simulink model "motor_param_persist"  (R2021a)
settings: configuration reference "motor_ctrl_config" (kept outside this file)
model workspace (MAT data in the model file):
  debounce = 4
  debounce_cnt_def = Simulink.Parameter
  debounce_cnt_def.Value = 0
  debounce_cnt_def.DataType = 'int16'
  debounce_cnt_def.Dimensions = [1 1]
values from neighbouring files (symbols this model uses):
  ee_ram = 1    [motor_ctrl_data.sldd]
undefined symbols (not defined in the file or in its folder): ee_commit
libraries: simulink x1
settings Model: DataDictionary=motor_ctrl_data.sldd  ParameterArgumentNames=debounce_cnt_def  OrderedModelArguments=off  Creator=Litao  LastModifiedBy=Litao
settings ConfigSetRef: SourceName=motor_ctrl_config

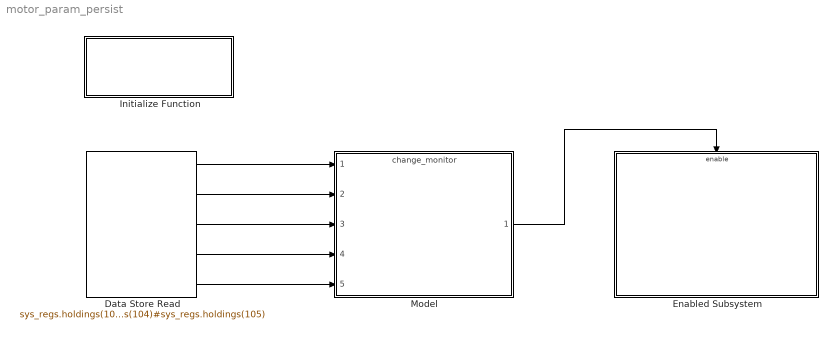
== system motor_param_persist ==
  Data Store Read : DataStoreRead  DataStoreName=sys_regs  DataStoreElements=sys_regs.holdings(101)#sys_regs.holdings(102)#sys_regs.holdings(103)#sys_regs.holdings(104)#sys_regs.holdings(105)  IndexOptions=Index vector (dialog)  Indices=1  OutputSizes=1
  Enabled Subsystem : Subsystem  TreatAsAtomicUnit=on
  Initialize Function : Subsystem  TreatAsAtomicUnit=on
  Model : ModelReference  ModelNameDialog=change_monitor.slx  SimulationMode=Normal  ModelReferenceVersion=1.14
  wires:
  Data Store Read/1 -> Model/1
  Data Store Read/2 -> Model/2
  Data Store Read/3 -> Model/3
  Data Store Read/4 -> Model/4
  Data Store Read/5 -> Model/5
  Model/1 -> Enabled Subsystem/Enable

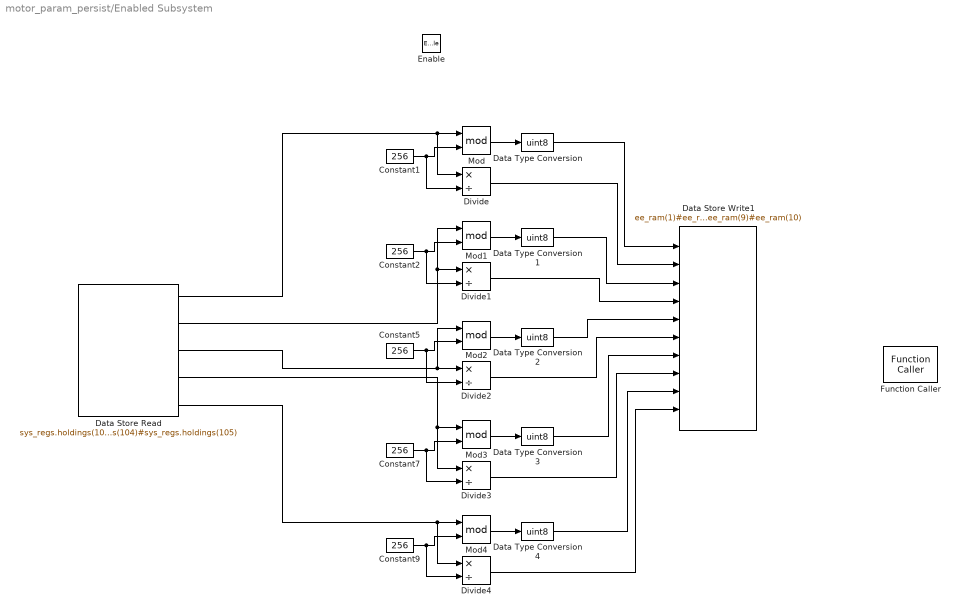
== system motor_param_persist/Enabled Subsystem ==
  Enable : EnablePort
  Constant{1..2,5,7,9} (5 alike) : Constant  Value=256  OutDataTypeStr=int16
  Data Store Read : DataStoreRead  DataStoreName=sys_regs  DataStoreElements=sys_regs.holdings(101)#sys_regs.holdings(102)#sys_regs.holdings(103)#sys_regs.holdings(104)#sys_regs.holdings(105)  IndexOptions=Index vector (dialog)  Indices=1  OutputSizes=1
  Data Store Write1 : DataStoreWrite  DataStoreName=ee_ram  DataStoreElements=ee_ram(1)#ee_ram(2)#ee_ram(3)#ee_ram(4)#ee_ram(5)#ee_ram(6)#ee_ram(7)#ee_ram(8)#ee_ram(9)#ee_ram(10)  IndexOptions=Index vector (dialog)  Indices=1  OutputSizes=1
  Data Type Conversion{,1..4} (5 alike) : DataTypeConversion  OutDataTypeStr=uint8
  Divide{,1..4} (5 alike) : Product  Inputs=*/  OutDataTypeStr=uint8
  Function Caller : FunctionCaller  FunctionPrototype=ee_commit()  InputArgumentSpecifications=<Enter example>  OutputArgumentSpecifications=<Enter example>
  Mod{,1..4} (5 alike) : Math  Operator=mod  OutputSignalType=real  SaturateOnIntegerOverflow=on
  wires:
  Divide4/1 -> Data Store Write1/10
  Data Type Conversion3/1 -> Data Store Write1/7
  Constant7/1 -> Divide3/2, Mod3/2
  Divide2/1 -> Data Store Write1/6
  Data Type Conversion2/1 -> Data Store Write1/5
  Data Store Read/3 -> Mod2/1, Divide2/1
  Data Store Read/5 -> Divide4/1, Mod4/1
  Constant5/1 -> Divide2/2, Mod2/2
  Data Type Conversion1/1 -> Data Store Write1/3
  Constant9/1 -> Divide4/2, Mod4/2
  Divide/1 -> Data Store Write1/2
  Mod4/1 -> Data Type Conversion4/1
  Constant2/1 -> Divide1/2, Mod1/2
  Data Store Read/4 -> Divide3/1, Mod3/1
  Mod3/1 -> Data Type Conversion3/1
  Divide1/1 -> Data Store Write1/4
  Constant1/1 -> Divide/2, Mod/2
  Data Store Read/2 -> Mod1/1, Divide1/1
  Divide3/1 -> Data Store Write1/8
  Data Store Read/1 -> Divide/1, Mod/1
  Mod2/1 -> Data Type Conversion2/1
  Data Type Conversion4/1 -> Data Store Write1/9
  Mod1/1 -> Data Type Conversion1/1
  Mod/1 -> Data Type Conversion/1
  Data Type Conversion/1 -> Data Store Write1/1

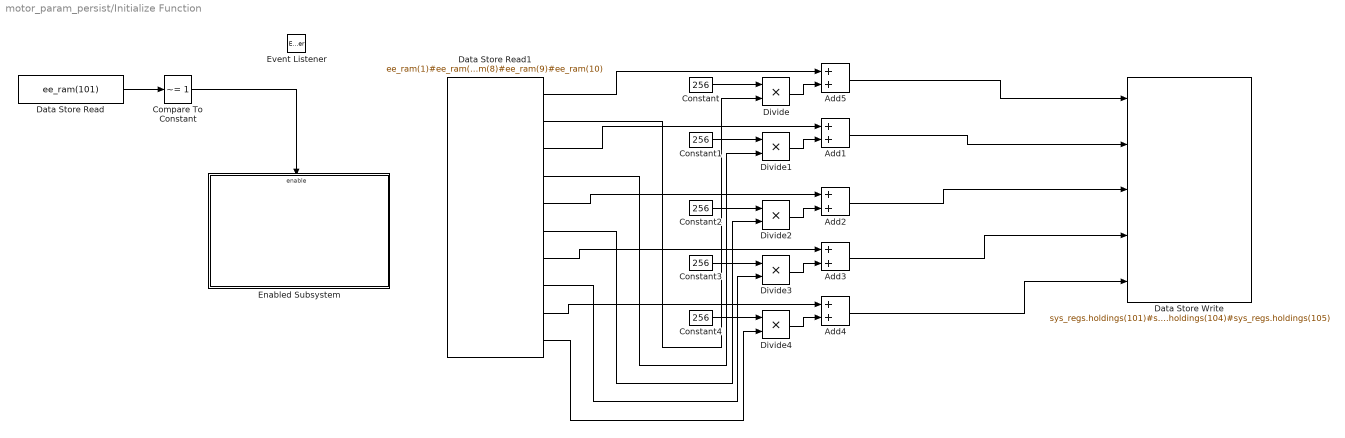
== system motor_param_persist/Initialize Function ==
  Add{1..5} (5 alike) : Sum  OutDataTypeStr=int16
  Compare To Constant : simulink/Logic and Bit Operations/Compare To Constant  relop=~=  const=1  OutDataTypeStr=boolean
  Constant{,1..4} (5 alike) : Constant  Value=256  OutDataTypeStr=int16
  Data Store Read : DataStoreRead  DataStoreName=ee_ram  DataStoreElements=ee_ram(101)  IndexOptions=Index vector (dialog)  Indices=1  OutputSizes=1
  Data Store Read1 : DataStoreRead  DataStoreName=ee_ram  DataStoreElements=ee_ram(1)#ee_ram(2)#ee_ram(3)#ee_ram(4)#ee_ram(5)#ee_ram(6)#ee_ram(7)#ee_ram(8)#ee_ram(9)#ee_ram(10)  IndexOptions=Index vector (dialog)  Indices=1  OutputSizes=1
  Data Store Write : DataStoreWrite  DataStoreName=sys_regs  DataStoreElements=sys_regs.holdings(101)#sys_regs.holdings(102)#sys_regs.holdings(103)#sys_regs.holdings(104)#sys_regs.holdings(105)  IndexOptions=Index vector (dialog)  Indices=1  OutputSizes=1
  Divide : Product  Inputs=**  OutDataTypeStr=int16
  Divide{1..4} (4 alike) : Product  Inputs=**
  Enabled Subsystem : Subsystem  TreatAsAtomicUnit=on
  Event Listener : EventListener  DisableCoverage=on  EventName=reset
  wires:
  Data Store Read/1 -> Compare To Constant/1
  Compare To Constant/1 -> Enabled Subsystem/Enable
  Add1/1 -> Data Store Write/2
  Constant4/1 -> Divide4/1
  Add4/1 -> Data Store Write/5
  Divide1/1 -> Add1/2
  Data Store Read1/8 -> Divide3/2
  Data Store Read1/5 -> Add2/1
  Data Store Read1/7 -> Add3/1
  Divide3/1 -> Add3/2
  Add2/1 -> Data Store Write/3
  Data Store Read1/9 -> Add4/1
  Data Store Read1/10 -> Divide4/2
  Constant3/1 -> Divide3/1
  Constant2/1 -> Divide2/1
  Data Store Read1/3 -> Add1/1
  Add5/1 -> Data Store Write/1
  Divide4/1 -> Add4/2
  Data Store Read1/6 -> Divide2/2
  Constant1/1 -> Divide1/1
  Divide2/1 -> Add2/2
  Data Store Read1/2 -> Divide/2
  Divide/1 -> Add5/2
  Add3/1 -> Data Store Write/4
  Data Store Read1/4 -> Divide1/2
  Data Store Read1/1 -> Add5/1
  Constant/1 -> Divide/1

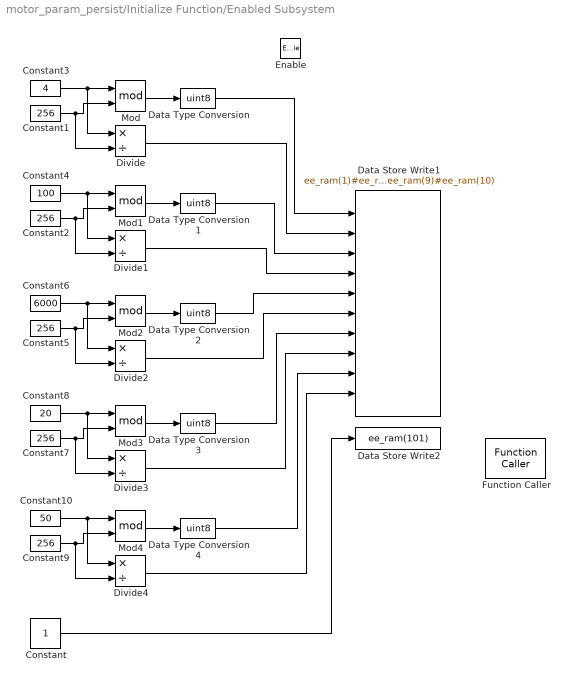
== system motor_param_persist/Initialize Function/Enabled Subsystem ==
  Enable : EnablePort
  Constant : Constant  OutDataTypeStr=uint8
  Constant{1..2,5,7,9} (5 alike) : Constant  Value=256  OutDataTypeStr=int16
  Constant10 : Constant  Value=50  OutDataTypeStr=int16
  Constant3 : Constant  Value=4  OutDataTypeStr=int16
  Constant4 : Constant  Value=100  OutDataTypeStr=int16
  Constant6 : Constant  Value=6000  OutDataTypeStr=int16
  Constant8 : Constant  Value=20  OutDataTypeStr=int16
  Data Store Write1 : DataStoreWrite  DataStoreName=ee_ram  DataStoreElements=ee_ram(1)#ee_ram(2)#ee_ram(3)#ee_ram(4)#ee_ram(5)#ee_ram(6)#ee_ram(7)#ee_ram(8)#ee_ram(9)#ee_ram(10)  IndexOptions=Index vector (dialog)  Indices=1  OutputSizes=1
  Data Store Write2 : DataStoreWrite  DataStoreName=ee_ram  DataStoreElements=ee_ram(101)  IndexOptions=Index vector (dialog)  Indices=1  OutputSizes=1
  Data Type Conversion{,1..4} (5 alike) : DataTypeConversion  OutDataTypeStr=uint8
  Divide{,1..4} (5 alike) : Product  Inputs=*/  OutDataTypeStr=uint8
  Function Caller : FunctionCaller  FunctionPrototype=ee_commit()  InputArgumentSpecifications=<Enter example>  OutputArgumentSpecifications=<Enter example>
  Mod{,1..4} (5 alike) : Math  Operator=mod  OutputSignalType=real  SaturateOnIntegerOverflow=on
  wires:
  Constant/1 -> Data Store Write2/1
  Constant3/1 -> Divide/1, Mod/1
  Constant1/1 -> Divide/2, Mod/2
  Mod/1 -> Data Type Conversion/1
  Data Type Conversion/1 -> Data Store Write1/1
  Divide/1 -> Data Store Write1/2
  Constant2/1 -> Divide1/2, Mod1/2
  Mod1/1 -> Data Type Conversion1/1
  Constant4/1 -> Divide1/1, Mod1/1
  Constant5/1 -> Divide2/2, Mod2/2
  Mod2/1 -> Data Type Conversion2/1
  Constant6/1 -> Divide2/1, Mod2/1
  Constant7/1 -> Divide3/2, Mod3/2
  Mod3/1 -> Data Type Conversion3/1
  Constant8/1 -> Divide3/1, Mod3/1
  Constant9/1 -> Divide4/2, Mod4/2
  Mod4/1 -> Data Type Conversion4/1
  Constant10/1 -> Divide4/1, Mod4/1
  Data Type Conversion1/1 -> Data Store Write1/3
  Divide1/1 -> Data Store Write1/4
  Data Type Conversion2/1 -> Data Store Write1/5
  Divide2/1 -> Data Store Write1/6
  Data Type Conversion3/1 -> Data Store Write1/7
  Divide3/1 -> Data Store Write1/8
  Data Type Conversion4/1 -> Data Store Write1/9
  Divide4/1 -> Data Store Write1/10
